simulink model "State_controller_first"  (Simulink 7.9)
settings: Solver=ode45  StartTime=0.0  StopTime=100.0  RelTol=1e-3
undefined symbols (not defined in the file or in its folder): sigbuilder_block
libraries: simulink x2
settings Model: Creator=dAN  LastModifiedBy=dAN

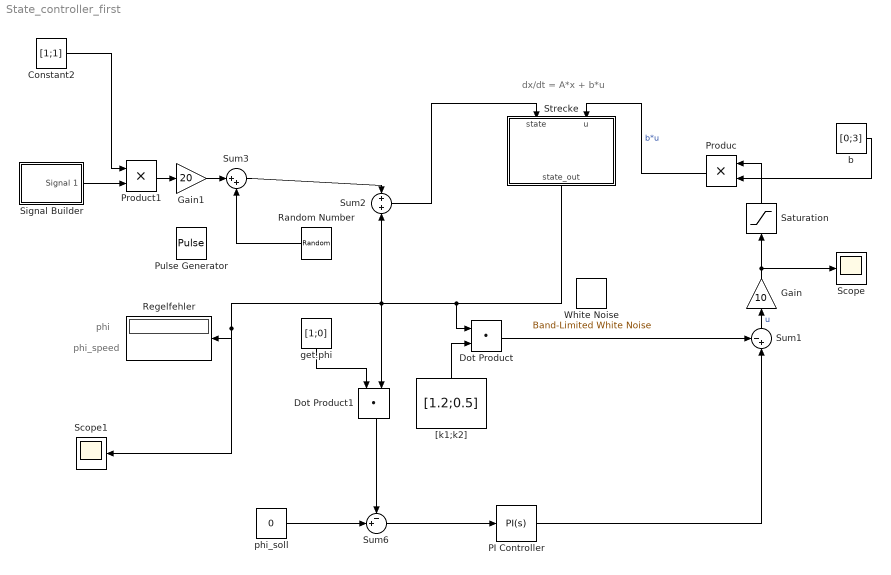
== system State_controller_first ==
  note: dx/dt = A*x + b*u
  note: phi_speed
  note: phi
  Constant2 : Constant  Value=[1;1]  VectorParams1D=off
  Dot Product : DotProduct  InputSameDT=on  OutDataTypeStr=Inherit: Inherit via internal rule
  Dot Product1 : DotProduct  InputSameDT=on  OutDataTypeStr=Inherit: Inherit via internal rule
  Gain : Gain  Gain=10
  Gain1 : Gain  Gain=20
  PI Controller : simulink/Continuous/PID Controller  Controller=PI  TimeDomain=Continuous-time  SampleTime=1  IntegratorMethod=Forward Euler  FilterMethod=Forward Euler  Form=Parallel  P=4  I=2  D=0  N=100  InitialConditionSource=internal  InitialConditionForIntegrator=0  InitialConditionForFilter=0  ExternalReset=none  LimitOutput=off  UpperSaturationLimit=inf  LowerSaturationLimit=-inf  LinearizeAsGain=off  AntiWindupMode=none  Kb=1  TrackingMode=off  Kt=1  PParamMin=[]  PParamMax=[]  IParamMin=[]  IParamMax=[]  DParamMin=[]  DParamMax=[]  NParamMin=[]  NParamMax=[]  KbParamMin=[]  KbParamMax=[]  KtParamMin=[]  KtParamMax=[]  POutMin=[]  POutMax=[]  IOutMin=[]  IOutMax=[]  DOutMin=[]  DOutMax=[]  NOutMin=[]  NOutMax=[]  KbOutMin=[]  KbOutMax=[]  KtOutMin=[]  KtOutMax=[]  IntegratorOutMin=[]  IntegratorOutMax=[]  FilterOutMin=[]  FilterOutMax=[]  SumOutMin=[]  SumOutMax=[]  SumI1OutMin=[]  SumI1OutMax=[]  SumI2OutMin=[]  SumI2OutMax=[]  SumI3OutMin=[]  SumI3OutMax=[]  SumDOutMin=[]  SumDOutMax=[]  SaturationOutMin=[]  SaturationOutMax=[]  IntegratorContinuousStateAttributes=''  IntegratorStateMustResolveToSignalObject=off  IntegratorRTWStateStorageClass=Auto  FilterContinuousStateAttributes=''  FilterStateMustResolveToSignalObject=off  FilterRTWStateStorageClass=Auto
  Produc : Product  RndMeth=Zero
  Product1 : Product  RndMeth=Zero
  Pulse Generator : DiscretePulseGenerator  PulseType=Time based  Amplitude=[5;5]  PulseWidth=5  VectorParams1D=off
  Random Number : UniformRandomNumber  Minimum=-[5;3]  Maximum=[5;3]  SampleTime=0.1  VectorParams1D=off
  Regelfehler : Display
  Saturation : Saturate  UpperLimit=45  LowerLimit=-45
  Scope : Scope
  Scope1 : Scope
      settings: TimeRange=100  YMin=-1  YMax=1
  Signal Builder : Subsystem  Tag=STV Subsys  LoadFcn=sigbuilder_block('load');  StartFcn=sigbuilder_block('start');  StopFcn=sigbuilder_block('stop');  ClipboardFcn=sigbuilder_block('clipboard');  mask(Sigbuilder block){}
      mask help: Simulink:masks:SigbuilderBlock_MD
      mask init:
      | if ~strcmp(get_param(bdroot(gcbh),'SimulationStatus'),'stopped') tuvar = sigbuilder_block('maskInit'); end
      settings: CopyFcn=sigbuilder_block('copy');  DeleteFcn=sigbuilder_block('delete');  ModelCloseFcn=sigbuilder_block('modelClose');  PreSaveFcn=sigbuilder_block('preSave');  PauseFcn=sigbuilder_block('pause');  ContinueFcn=sigbuilder_block('continue');  NameChangeFcn=sigbuilder_block('namechange');  OpenFcn=sigbuilder_block('open',[437.25 199.5 550.5 399.75 ]);  CloseFcn=sigbuilder_block('close');
      mask Display: plot(0, 0, 100, 100,[2, 2, 32, 32, 2], [68, 8, 8, 68, 68],[32, 2], [38, 38], [32, 19, 2],[53, 60, 44], [32, 17, 17, 2],[16, 16, 31, 31]);txt = getActiveGroup(gcbh);text(2, 100, txt,'verticalAlignment', 'top');
  Strecke : Subsystem
  Sum1 : Sum  Inputs=-+|
  Sum2 : Sum
  Sum3 : Sum  Inputs=|++
  Sum6 : Sum  Inputs=-+|
  White Noise : simulink/Sources/Band-Limited White Noise  Cov=[0.1]  Ts=0.1  seed=[23341]  VectorParams1D=off
  "[k1;k2]" : Constant  Value=[1.2;0.5]  VectorParams1D=off
  b : Constant  Value=[0;3]  VectorParams1D=off
  get.phi : Constant  Value=[1;0]  VectorParams1D=off
  phi_soll : Constant  Value=0  VectorParams1D=off
  wires:
  Sum1/1 -> Gain/1  "u"
  "[k1;k2]"/1 -> Dot Product/2
  Dot Product/1 -> Sum1/1
  b/1 -> Produc/2
  Sum2/1 -> Strecke/1(state)
  Dot Product1/1 -> Sum6/1
  Sum3/1 -> Sum2/1
  Gain1/1 -> Sum3/1
  Product1/1 -> Gain1/1
  Constant2/1 -> Product1/1
  get.phi/1 -> Dot Product1/1
  phi_soll/1 -> Sum6/2
  Signal Builder/1(Signal 1) -> Product1/2
  Produc/1 -> Strecke/2(u)  "b*u"
  Strecke/1(state_out) -> Dot Product/1, Sum2/2, Dot Product1/2, Regelfehler/1, Scope1/1
  Sum6/1 -> PI Controller/1
  Random Number/1 -> Sum3/2
  Saturation/1 -> Produc/1
  Gain/1 -> Saturation/1, Scope/1
  PI Controller/1 -> Sum1/2

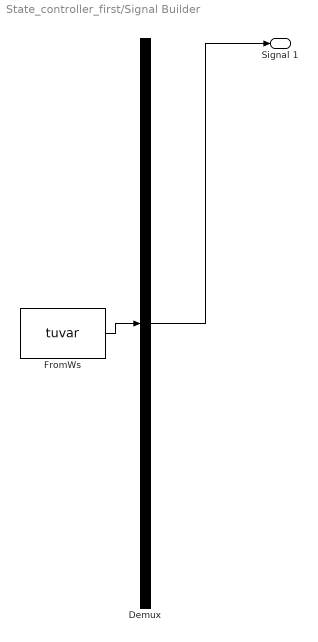
== system State_controller_first/Signal Builder ==
  Demux : Demux  Tag=STV Demux  Outputs=1
  FromWs : FromWorkspace  Tag=STV FromWs  VariableName=tuvar  SampleTime=0  SigBuilderData=DataTag0  VnvData=DataTag1
      SigBuilderData=|
      | common.afterFinalStr = 'Extrapolate'
      | common.sampleTime = 0
      | dataSet.timeRange = [0 10]
      | dataSet.name = 'Group 1'
      | sbobj.Groups.Name = 'Group 1'
      | sbobj.Groups.Signals.Name = 'Signal 1'
      | sbobj.Groups.Signals.XData = [0 4 4 6 6 10]
      | sbobj.Groups.Signals.YData = [0 0 1 1 0.005 0.005]
  Signal 1 : Outport  Tag=STV Outport
  wires:
  Demux/1 -> Signal 1/1
  FromWs/1 -> Demux/1

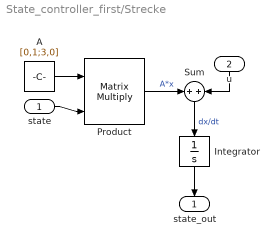
== system State_controller_first/Strecke ==
  state : Inport
  u : Inport  Port=2
  A : Constant  Value=[0,1;3,0]  VectorParams1D=off
  Integrator : Integrator  LimitOutput=on  UpperSaturationLimit=90  LowerSaturationLimit=-90
  Product : Product  Multiplication=Matrix(*)  RndMeth=Zero
  Sum : Sum
  state_out : Outport
  wires:
  A/1 -> Product/1
  Product/1 -> Sum/1  "A*x"
  u/1 -> Sum/2
  state/1 -> Product/2
  Sum/1 -> Integrator/1  "dx/dt"
  Integrator/1 -> state_out/1
